simulink model "MDL1_Longitudinal_Vehicle_Model"  (R2025b)
settings: Solver=VariableStepAuto  StartTime=0.0  StopTime=20  MaxStep=1/100  MinStep=1/1000  RelTol=1e-3
InitFcn:
  | mdl1_longitudinal_vehicle_init_params
undefined symbols (not defined in the file): A, C_d, F_T, g, m, rho, theta, v
settings Model: Creator=rkash  LastModifiedBy=rkash

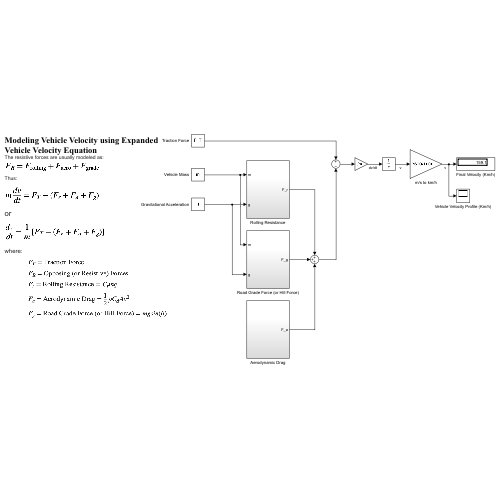
[thumbnail: Simulink's stored preview of the top-level diagram]
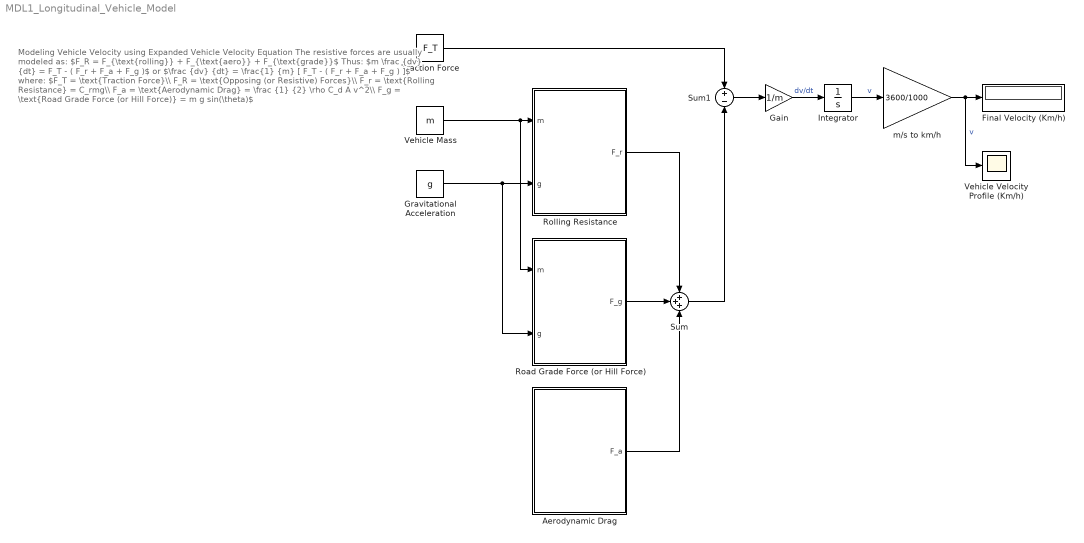
== system MDL1_Longitudinal_Vehicle_Model ==
  note: Modeling Vehicle Velocity using Expanded Vehicle Velocity Equation
      | The resistive forces are usually modeled as:
      | $F_R = F_{\text{rolling}} + F_{\text{aero}} + F_{\text{grade}}$
      | Thus:
      | $m \frac {dv} {dt} = F_T - ( F_r + F_a + F_g )$
      | or
      | $\frac {dv} {dt} = \frac{1} {m} [ F_T - ( F_r + F_a + F_g ) ]$
      | where:
      | $F_T = \text{Traction Force}\\ F_R = \text{Opposing (or Resistive) Forces}\\ F_r = \text{Rolling Resistance} = C_rmg\\ F_a = \text{Aerodynamic Drag} = \frac {1} {2} \rho C_d A v^2\\ F_g = \text{Road Grade Force (or Hill Force)} = m g sin(\theta)$
  Aerodynamic Drag : Subsystem
  Final Velocity (Km/h) : Display
  Gain : Gain  Gain=1/m
  Gravitational Acceleration : Constant  Value=g
  Integrator : Integrator
  Road Grade Force (or Hill Force) : Subsystem
  Rolling Resistance : Subsystem
  Sum : Sum  Inputs=+++
  Sum1 : Sum  Inputs=+-
  Traction Force : Constant  Value=F_T
  Vehicle Mass : Constant  Value=m
  Vehicle Velocity Profile (Km/h) : Scope
      settings: ActiveDisplayYMinimum=-19.882049999999989  ActiveDisplayYMaximum=178.93844999999993
  m/s to km/h : Gain  Gain=3600/1000
  wires:
  Vehicle Mass/1 -> Rolling Resistance/1(m), Road Grade Force (or Hill Force)/1(m)
  Gravitational Acceleration/1 -> Rolling Resistance/2(g), Road Grade Force (or Hill Force)/2(g)
  Rolling Resistance/1(F_r) -> Sum/1
  Road Grade Force (or Hill Force)/1(F_g) -> Sum/2
  Aerodynamic Drag/1(F_a) -> Sum/3
  Traction Force/1 -> Sum1/1
  Sum/1 -> Sum1/2
  Sum1/1 -> Gain/1
  Gain/1 -> Integrator/1  "dv/dt"
  Integrator/1 -> m/s to km/h/1  "v"
  m/s to km/h/1 -> Vehicle Velocity Profile (Km/h)/1, Final Velocity (Km/h)/1  "v"

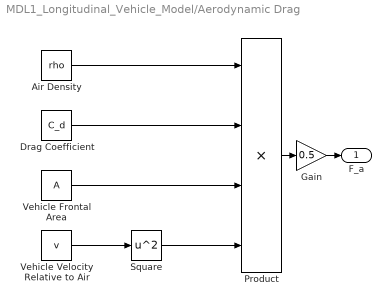
== system MDL1_Longitudinal_Vehicle_Model/Aerodynamic Drag ==
  Air Density : Constant  Value=rho
  Drag Coefficient : Constant  Value=C_d
  Gain : Gain  Gain=0.5
  Product : Product  Inputs=4
  Square : Math  Operator=square
  Vehicle Frontal Area : Constant  Value=A
  Vehicle Velocity Relative to Air : Constant  Value=v
  F_a : Outport
  wires:
  Vehicle Frontal Area/1 -> Product/3
  Drag Coefficient/1 -> Product/2
  Air Density/1 -> Product/1
  Product/1 -> Gain/1
  Gain/1 -> F_a/1
  Vehicle Velocity Relative to Air/1 -> Square/1
  Square/1 -> Product/4

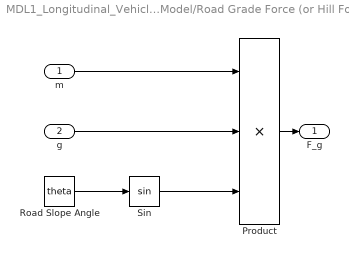
== system MDL1_Longitudinal_Vehicle_Model/Road Grade Force (or Hill Force) ==
  m : Inport
  g : Inport  Port=2
  Product : Product  Inputs=3
  Road Slope Angle : Constant  Value=theta
  Sin : Trigonometry
  F_g : Outport
  wires:
  m/1 -> Product/1
  g/1 -> Product/2
  Product/1 -> F_g/1
  Sin/1 -> Product/3
  Road Slope Angle/1 -> Sin/1

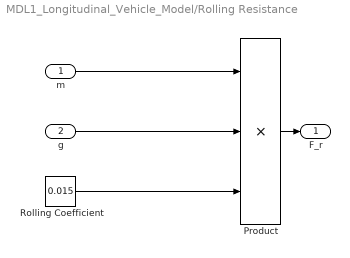
== system MDL1_Longitudinal_Vehicle_Model/Rolling Resistance ==
  m : Inport
  g : Inport  Port=2
  Product : Product  Inputs=3
  Rolling Coefficient : Constant  Value=0.015
  F_r : Outport
  wires:
  Rolling Coefficient/1 -> Product/3
  Product/1 -> F_r/1
  g/1 -> Product/2
  m/1 -> Product/1
